simulink model "sampleModel1764"  (R2023a)
settings: Solver=VariableStepAuto  StartTime=0.0  StopTime=10.0  RelTol=1e-3
libraries: simulink x4, hdlsllib x2
settings Model: Creator=user1  LastModifiedBy=user1

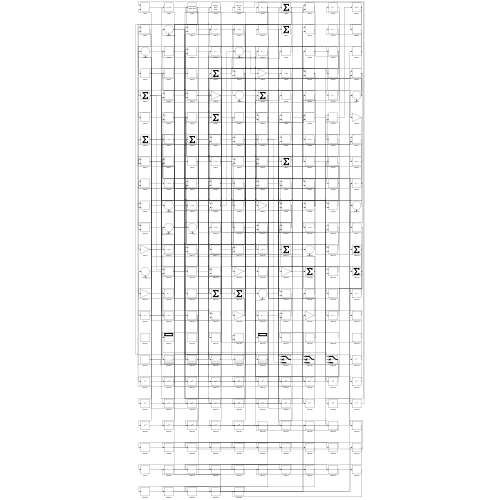
[thumbnail: Simulink's stored preview of the top-level diagram]
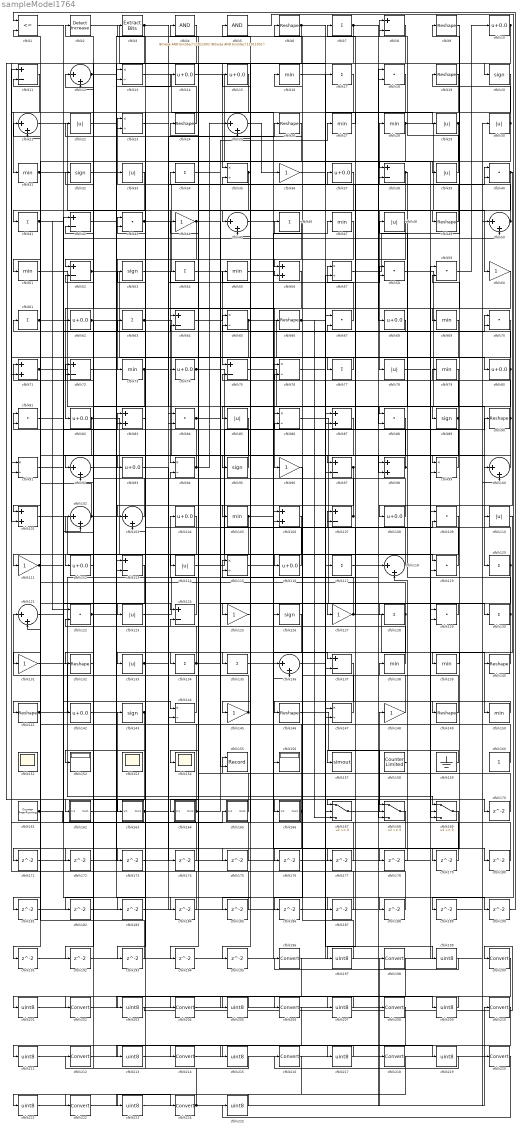
== system sampleModel1764 ==
  cfblk1 : RelationalOperator  Operator=<=  OutDataTypeStr=boolean  InputSameDT=off
  cfblk{10,14..15,37,62,68,74,80,82,93,104,108,112,116,142} (15 alike) : Bias  Bias=0.0  SaturateOnIntegerOverflow=off
  cfblk{12,21,25,45,50,92,100,102..103,118,121,136} (12 alike) : Sum  Inputs=|++
  cfblk{56,71,83,87,98,101,106} (7 alike) : Sum
  cfblk{16,27..28,31,47,51,55,69,73,79,105,138..139,150} (14 alike) : MinMax
  cfblk{8,11,38,42,52,64,72,75,97,107,113,124,137} (13 alike) : Sum  Inputs=+-
  cfblk{18,40,43,58..59,67,70,81,84,88,109,119,122,129} (14 alike) : DotProduct  OutDataTypeStr=Inherit: Inherit via internal rule
  cfblk{22,29..30,33,39,48,78,85,110,114,123,133} (12 alike) : Abs  SaturateOnIntegerOverflow=off
  cfblk{36,44,60,96,111,125,127,131,145,148} (10 alike) : Gain
  cfblk{13,23,35,57,65,76,86,91,94,99,115,144,147} (13 alike) : Product  Inputs=*/  RndMeth=Zero  SaturateOnIntegerOverflow=on
  cfblk{7,17,34,41,46,54,61,63,77,117,120,128,130,134..135} (15 alike) : Sum  Inputs=+
  cfblk{20,32,53,89,95,126,143} (7 alike) : Signum
  cfblk{6,9,19,24,26,49,66,90,132,140..141,146,149} (13 alike) : Reshape
  cfblk151 : Scope
      settings: Floating=on
  cfblk152 : Display
  cfblk153 : Scope
      settings: Floating=on
  cfblk154 : Scope
  cfblk155 : Record  FileSettingsInternal="{\"entries\":[{\"content\":{\"excelSettings\":{\"content\":{},\"type\":\"Streamout.ExcelSettings\"}},\"type\":\"Streamout.FileSettingStorage\",\"uuid\":\"\"}],\"packageUris\":[\"http:\\/\\/schema.mathworks.com\\/mf0\\/streamout_blocks\\/R2020a\"],\"version\":\"1.0\"}"  Layout=[1 1]  SignalsInternal="{\"entries\":[{\"content\":{\"signals\":[{\"content\":{\"blockPath\":[],\"dimensions\":[1],\"domain\":\"\",\"lineColor\":\"#a2142f\",\"plots\":[1],\"port\":1,\"signalID\":3838,\"signalName\":\"XY Graph:1\"},\"type\":\"RecordBlkView.Signal\",\"uuid\":\"\"},{\"content\":{\"blockPath\":[],\"dimensions\":[1],\"domain\":\"\",\"lineColor\":\"#139fff\",\"plots\":[1],\"port\":2,\"signalID\":3841,\"signalName\":\"XY Graph:2\"},\"type\":\"RecordBlkView.Signal\",\"uuid\":\"\"}]},\"type\":\"RecordBlkView.InputSignals\",\"uuid\":\"\"}],\"packageUris\":[\"http:\\/\\/schema.mathworks.com\\/mf0\\/streamout_blocks\\/R2020a\"],\"version\":\"1.0\"}"  VisualizationBindings="{\"xyplotplugin\":{\"info\":[{\"series\":[{\"bindingParametersList\":[{\"parameter\":\"X-Axis\",\"signalID\":3838,\"signalName\":\"XY Graph:1\"},{\"parameter\":\"Y-Axis\",\"signalID\":3841,\"signalName\":\"XY Graph:2\"}],\"seriesID\":10623}],\"subplotID\":1}]}}"  CompatibilityTag=XY  st=-1
  cfblk156 : Display
  cfblk157 : ToWorkspace  VariableName=simout  SaveFormat=Timeseries  SampleTime=-1
  cfblk158 : hdlsllib/Sources/Counter Limited  uplimit=7  tsamp=-1
  cfblk159 : Ground
  cfblk160 : Constant  SampleTime=-1
  cfblk161 : hdlsllib/Sources/Counter Free-Running  NumBits=16  tsamp=-1
  cfblk162 : Subsystem
      settings: LibrarySourceBlock=|
      | hdlsllib/Ports &
      | Subsystems/Subsystem
  cfblk163 : Subsystem
      settings: LibrarySourceBlock=|
      | hdlsllib/Ports &
      | Subsystems/Subsystem
  cfblk164 : Subsystem
      settings: LibrarySourceBlock=|
      | hdlsllib/Ports &
      | Subsystems/Subsystem
  cfblk165 : Subsystem
      settings: LibrarySourceBlock=|
      | hdlsllib/Ports &
      | Subsystems/Subsystem
  cfblk166 : Subsystem
      settings: LibrarySourceBlock=|
      | hdlsllib/Ports &
      | Subsystems/Subsystem
  cfblk167 : Switch  SaturateOnIntegerOverflow=off  InputSameDT=off
  cfblk168 : Switch  SaturateOnIntegerOverflow=off  InputSameDT=off
  cfblk169 : Switch  SaturateOnIntegerOverflow=off  InputSameDT=off
  cfblk{170..195} (26 alike) : Delay  SampleTime=1
  cfblk{196,198,200,202,204,206,208,210,212,214,216,218,220,222,224} (15 alike) : DataTypeConversion  SaturateOnIntegerOverflow=off  RndMeth=Floor
  cfblk{197,199,201,203,205,207,209,211,213,215,217,219,221,223,225} (15 alike) : DataTypeConversion  OutDataTypeStr=uint8  SaturateOnIntegerOverflow=off  RndMeth=Floor
  cfblk2 : simulink/Logic and Bit Operations/Detect Increase  vinit=0.0  OutDataTypeStr=boolean
      settings: LibrarySourceBlock=|
      | hdlsllib/Logic and Bit
      | Operations/Detect
      | Increase
  cfblk3 : simulink/Logic and Bit Operations/Extract Bits  bitsToExtract=Upper half  numBits=8  bitIdxRange=[0 7]  outScalingMode=Preserve fixed-point scaling
      settings: LibrarySourceBlock=|
      | hdlsllib/Logic and Bit
      | Operations/Extract Bits
  cfblk4 : simulink/Logic and Bit Operations/Bitwise Operator  logicop=AND  UseBitMask=on  BitMask=bin2dec('11011001')  BitMaskRealWorld=Stored Integer
      settings: LibrarySourceBlock=|
      | hdlsllib/Logic and Bit
      | Operations/Bitwise
      | Operator
  cfblk5 : simulink/Logic and Bit Operations/Bitwise Operator  logicop=AND  UseBitMask=on  BitMask=bin2dec('11011001')  BitMaskRealWorld=Stored Integer
      settings: LibrarySourceBlock=|
      | hdlsllib/Logic and Bit
      | Operations/Bitwise
      | Operator
  wires:
  cfblk159/1 -> cfblk157/1
  cfblk129/1 -> cfblk125/1
  cfblk103/1 -> cfblk71/1
  cfblk124/1 -> cfblk104/1
  cfblk12/1 -> cfblk187/1, cfblk188/1
  cfblk89/1 -> cfblk15/1, cfblk175/1
  cfblk43/1 -> cfblk49/1, cfblk66/1
  cfblk57/1 -> cfblk19/1
  cfblk99/1 -> cfblk37/1
  cfblk87/1 -> cfblk112/1
  cfblk138/1 -> cfblk34/1
  cfblk75/1 -> cfblk89/1
  cfblk59/1 -> cfblk10/1
  cfblk52/1 -> cfblk80/1, cfblk184/1
  cfblk24/1 -> cfblk162/1(In1)
  cfblk82/1 -> cfblk119/1, cfblk121/2
  cfblk101/1 -> cfblk116/1
  cfblk49/1 -> cfblk23/1
  cfblk92/1 -> cfblk156/1
  cfblk15/1 -> cfblk91/2
  cfblk131/1 -> cfblk169/1
  cfblk48/1 -> cfblk167/1
  cfblk60/1 -> cfblk96/1
  cfblk28/1 -> cfblk60/1, cfblk177/1
  cfblk21/1 -> cfblk94/1
  cfblk86/1 -> cfblk130/1
  cfblk25/1 -> cfblk36/1
  cfblk19/1 -> cfblk133/1
  cfblk67/1 -> cfblk57/1
  cfblk80/1 -> cfblk65/2, cfblk185/1
  cfblk3/1 -> cfblk52/1, cfblk12/2, cfblk87/2
  cfblk160/1 -> cfblk1/2
  cfblk31/1 -> cfblk78/1, cfblk98/2
  cfblk141/1 -> cfblk33/1, cfblk63/1
  cfblk6/1 -> cfblk35/1, cfblk29/1, cfblk71/2
  cfblk35/1 -> cfblk45/1, cfblk85/1
  cfblk40/1 -> cfblk108/1, cfblk74/1
  cfblk144/1 -> cfblk121/1
  cfblk167/1 -> cfblk148/1
  cfblk117/1 -> cfblk18/1
  cfblk58/1 -> cfblk120/1
  cfblk11/1 -> cfblk31/1
  cfblk134/1 -> cfblk24/1, cfblk72/2, cfblk27/1, cfblk103/2
  cfblk111/1 -> cfblk102/2, cfblk83/1
  cfblk56/1 -> cfblk82/1
  cfblk143/1 -> cfblk152/1, cfblk172/1
  cfblk13/1 -> cfblk136/1
  cfblk97/1 -> cfblk145/1, cfblk173/1
  cfblk53/1 -> cfblk17/1
  cfblk18/1 -> cfblk106/2
  cfblk14/1 -> cfblk129/1
  cfblk50/1 -> cfblk28/1, cfblk6/1
  cfblk7/1 -> cfblk68/1, cfblk43/2, cfblk64/1
  cfblk34/1 -> cfblk38/1
  cfblk47/1 -> cfblk73/1
  cfblk68/1 -> cfblk67/2
  cfblk38/1 -> cfblk88/1, cfblk135/1
  cfblk116/1 -> cfblk61/1
  cfblk130/1 -> cfblk149/1, cfblk76/2, cfblk179/1
  cfblk107/1 -> cfblk46/1, cfblk103/1
  cfblk162/1(Out1) -> cfblk143/1
  cfblk109/1 -> cfblk111/1
  cfblk161/1 -> cfblk165/1(In1), cfblk64/2
  cfblk74/1 -> cfblk119/2, cfblk99/1
  cfblk46/1 -> cfblk56/1
  cfblk166/1(Out1) -> cfblk115/2, cfblk182/1
  cfblk149/1 -> cfblk81/1
  cfblk32/1 -> cfblk23/2
  cfblk65/1 -> cfblk123/1, cfblk87/1
  cfblk113/1 -> cfblk141/1
  cfblk158/1 -> cfblk138/1
  cfblk30/1 -> cfblk101/1, cfblk9/1
  cfblk63/1 -> cfblk169/2, cfblk40/1
  cfblk29/1 -> cfblk114/1, cfblk51/1
  cfblk83/1 -> cfblk43/1
  cfblk61/1 -> cfblk110/1, cfblk99/2
  cfblk9/1 -> cfblk69/1
  cfblk139/1 -> cfblk79/1
  cfblk10/1 -> cfblk20/1, cfblk25/2
  cfblk120/1 -> cfblk59/2, cfblk154/1
  cfblk147/1 -> cfblk22/1
  cfblk20/1 -> cfblk97/1
  cfblk119/1 -> cfblk5/1
  cfblk150/1 -> cfblk146/1
  cfblk23/1 -> cfblk39/1
  cfblk127/1 -> cfblk150/1, cfblk107/2, cfblk35/2
  cfblk114/1 -> cfblk90/1
  cfblk135/1 -> cfblk137/1
  cfblk100/1 -> cfblk95/1
  cfblk62/1 -> cfblk86/1, cfblk192/1
  cfblk90/1 -> cfblk163/1(In1), cfblk55/1
  cfblk125/1 -> cfblk45/2
  cfblk42/1 -> cfblk13/2
  cfblk88/1 -> cfblk131/1
  cfblk44/1 -> cfblk93/1, cfblk127/1
  cfblk165/1(Out1) -> cfblk155/1
  cfblk115/1 -> cfblk47/1
  cfblk22/1 -> cfblk166/1(In1)
  cfblk163/1(Out1) -> cfblk84/1, cfblk70/1
  cfblk112/1 -> cfblk12/1
  cfblk95/1 -> cfblk11/2
  cfblk33/1 -> cfblk41/1
  cfblk84/1 -> cfblk4/1, cfblk128/1
  cfblk73/1 -> cfblk92/1, cfblk3/1, cfblk26/1, cfblk183/1
  cfblk81/1 -> cfblk142/1
  cfblk8/1 -> cfblk105/1
  cfblk72/1 -> cfblk88/2
  cfblk123/1 -> cfblk38/2
  cfblk2/1 -> cfblk117/1
  cfblk108/1 -> cfblk32/1
  cfblk71/1 -> cfblk155/2, cfblk144/2, cfblk191/1
  cfblk148/1 -> cfblk86/2
  cfblk79/1 -> cfblk167/2
  cfblk94/1 -> cfblk2/1, cfblk25/1
  cfblk132/1 -> cfblk92/2
  cfblk69/1 -> cfblk101/2
  cfblk106/1 -> cfblk134/1
  cfblk110/1 -> cfblk140/1
  cfblk91/1 -> cfblk50/2
  cfblk55/1 -> cfblk56/2
  cfblk104/1 -> cfblk113/2
  cfblk105/1 -> cfblk180/1, cfblk181/1
  cfblk26/1 -> cfblk164/1(In1)
  cfblk146/1 -> cfblk168/1
  cfblk85/1 -> cfblk132/1
  cfblk133/1 -> cfblk58/1, cfblk40/2
  cfblk118/1 -> cfblk54/1
  cfblk70/1 -> cfblk77/1
  cfblk128/1 -> cfblk81/2, cfblk193/1
  cfblk102/1 -> cfblk21/1, cfblk14/1, cfblk168/3, cfblk70/2
  cfblk78/1 -> cfblk169/3
  cfblk1/1 -> cfblk124/1
  cfblk140/1 -> cfblk139/1
  cfblk54/1 -> cfblk75/1
  cfblk98/1 -> cfblk42/2, cfblk83/2, cfblk48/1
  cfblk77/1 -> cfblk76/1
  cfblk36/1 -> cfblk129/2
  cfblk66/1 -> cfblk58/2, cfblk167/3
  cfblk27/1 -> cfblk7/1
  cfblk39/1 -> cfblk8/1
  cfblk122/1 -> cfblk115/1, cfblk144/1
  cfblk76/1 -> cfblk147/2
  cfblk136/1 -> cfblk109/2
  cfblk51/1 -> cfblk126/1
  cfblk37/1 -> cfblk137/2
  cfblk164/1(Out1) -> cfblk52/2, cfblk107/1
  cfblk145/1 -> cfblk72/1, cfblk44/1
  cfblk142/1 -> cfblk8/2
  cfblk4/1 -> cfblk62/1
  cfblk41/1 -> cfblk100/1, cfblk122/1, cfblk170/1
  cfblk64/1 -> cfblk65/1
  cfblk170/1 -> cfblk124/2
  cfblk169/1 -> cfblk171/1
  cfblk171/1 -> cfblk113/1
  cfblk172/1 -> cfblk106/1
  cfblk173/1 -> cfblk18/2
  cfblk93/1 -> cfblk174/1
  cfblk174/1 -> cfblk42/1
  cfblk175/1 -> cfblk11/1
  cfblk96/1 -> cfblk176/1
  cfblk176/1 -> cfblk109/1
  cfblk177/1 -> cfblk75/2
  cfblk45/1 -> cfblk178/1
  cfblk178/1 -> cfblk118/2
  cfblk179/1 -> cfblk13/1
  cfblk180/1 -> cfblk98/1
  cfblk181/1 -> cfblk168/2
  cfblk182/1 -> cfblk147/1
  cfblk183/1 -> cfblk84/2
  cfblk184/1 -> cfblk91/1
  cfblk185/1 -> cfblk102/1
  cfblk137/1 -> cfblk186/1
  cfblk186/1 -> cfblk57/2
  cfblk187/1 -> cfblk67/1
  cfblk188/1 -> cfblk94/2
  cfblk5/1 -> cfblk189/1
  cfblk189/1 -> cfblk50/1
  cfblk121/1 -> cfblk190/1
  cfblk190/1 -> cfblk1/1
  cfblk191/1 -> cfblk100/2
  cfblk192/1 -> cfblk136/2
  cfblk193/1 -> cfblk21/2
  cfblk126/1 -> cfblk194/1
  cfblk194/1 -> cfblk97/2
  cfblk17/1 -> cfblk195/1
  cfblk195/1 -> cfblk59/1
  cfblk168/1 -> cfblk197/1
  cfblk197/1 -> cfblk16/1
  cfblk16/1 -> cfblk199/1
  cfblk199/1 -> cfblk196/1
  cfblk196/1 -> cfblk201/1
  cfblk201/1 -> cfblk198/1
  cfblk198/1 -> cfblk203/1
  cfblk203/1 -> cfblk200/1
  cfblk200/1 -> cfblk205/1
  cfblk205/1 -> cfblk202/1
  cfblk202/1 -> cfblk207/1
  cfblk207/1 -> cfblk204/1
  cfblk204/1 -> cfblk209/1
  cfblk209/1 -> cfblk206/1
  cfblk206/1 -> cfblk211/1
  cfblk211/1 -> cfblk208/1
  cfblk208/1 -> cfblk213/1
  cfblk213/1 -> cfblk210/1
  cfblk210/1 -> cfblk215/1
  cfblk215/1 -> cfblk212/1
  cfblk212/1 -> cfblk217/1
  cfblk217/1 -> cfblk214/1
  cfblk214/1 -> cfblk219/1
  cfblk219/1 -> cfblk216/1
  cfblk216/1 -> cfblk221/1
  cfblk221/1 -> cfblk218/1
  cfblk222/1 -> cfblk224/1
  cfblk218/1 -> cfblk223/1
  cfblk223/1 -> cfblk220/1
  cfblk224/1 -> cfblk122/2, cfblk53/1, cfblk30/1, cfblk118/1
  cfblk220/1 -> cfblk225/1
  cfblk225/1 -> cfblk222/1

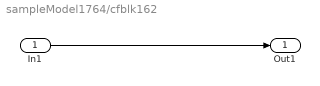
== system sampleModel1764/cfblk162 ==
  In1 : Inport
  Out1 : Outport
  wires:
  In1/1 -> Out1/1

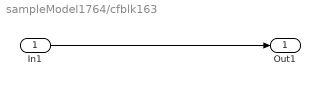
== system sampleModel1764/cfblk163 ==
  In1 : Inport
  Out1 : Outport
  wires:
  In1/1 -> Out1/1

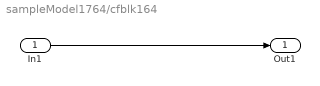
== system sampleModel1764/cfblk164 ==
  In1 : Inport
  Out1 : Outport
  wires:
  In1/1 -> Out1/1

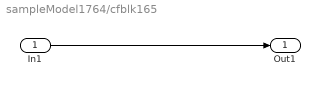
== system sampleModel1764/cfblk165 ==
  In1 : Inport
  Out1 : Outport
  wires:
  In1/1 -> Out1/1

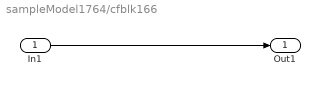
== system sampleModel1764/cfblk166 ==
  In1 : Inport
  Out1 : Outport
  wires:
  In1/1 -> Out1/1
